simulink model "first_gear_model_non_linear"  (R2020b)
settings: Solver=FixedStepAuto  StartTime=0.0  StopTime=5  FixedStep=0.0001  RelTol=1e-3
settings Model: Creator=morro  LastModifiedBy=morro

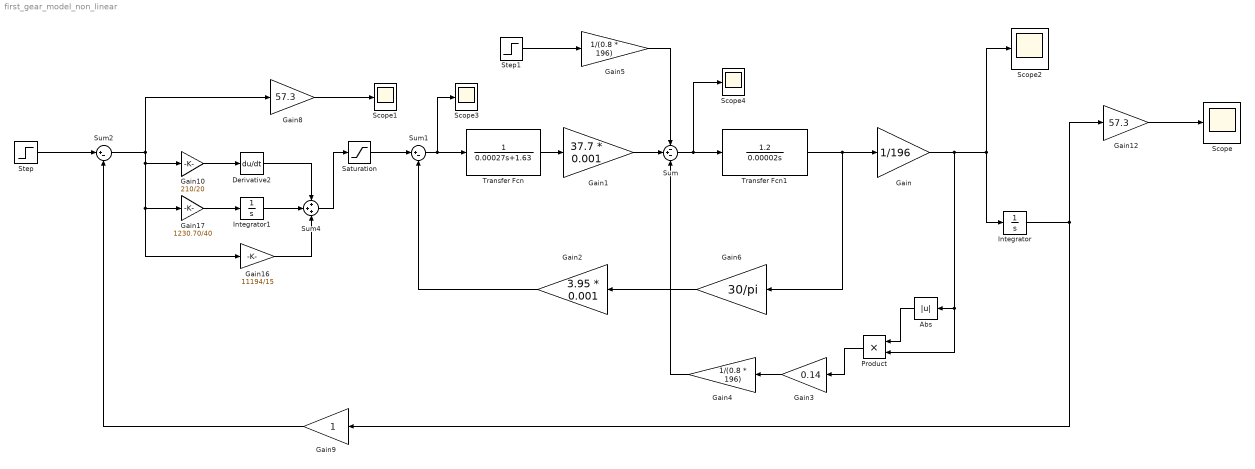
== system first_gear_model_non_linear ==
  Abs : Abs
  Derivative2 : Derivative
  Gain : Gain  Gain=1/196
  Gain1 : Gain  Gain=37.7 * 0.001
  Gain10 : Gain  Gain=210/20
  Gain12 : Gain  Gain=57.3
  Gain16 : Gain  Gain=11194/15
  Gain17 : Gain  Gain=1230.70/40
  Gain2 : Gain  Gain=3.95 * 0.001
  Gain3 : Gain  Gain=0.14
  Gain4 : Gain  Gain=1/(0.8 * 196)
  Gain5 : Gain  Gain=1/(0.8 * 196)
  Gain6 : Gain  Gain=30/pi
  Gain8 : Gain  Gain=57.3
  Gain9 : Gain
  Integrator : Integrator  InitialCondition=1e-7
  Integrator1 : Integrator  InitialCondition=1e-7
  Product : Product
  Saturation : Saturate  UpperLimit=27  LowerLimit=-27
  Scope{,1..4} (5 alike) : Scope
  Step : Step  After=100/57.3  SampleTime=0
  Step1 : Step  Time=2  After=9  SampleTime=0
  Sum : Sum  Inputs=-+-
  Sum1 : Sum  Inputs=|+-
  Sum2 : Sum  Inputs=|+-
  Sum4 : Sum  Inputs=+++
  Transfer Fcn : TransferFcn  Denominator=[0.00027 1.63]
  Transfer Fcn1 : TransferFcn  Numerator=[1.2]  Denominator=[0.00002 0]
  wires:
  Gain/1 -> Product/2, Abs/1, Integrator/1, Scope2/1
  Gain3/1 -> Gain4/1
  Gain9/1 -> Sum2/2
  Transfer Fcn/1 -> Gain1/1
  Integrator1/1 -> Sum4/2
  Gain17/1 -> Integrator1/1
  Gain2/1 -> Sum1/2
  Abs/1 -> Product/1
  Gain12/1 -> Scope/1
  Sum2/1 -> Gain16/1, Gain17/1, Gain10/1, Gain8/1
  Derivative2/1 -> Sum4/1
  Gain5/1 -> Sum/1
  Gain8/1 -> Scope1/1
  Step/1 -> Sum2/1
  Gain6/1 -> Gain2/1
  Transfer Fcn1/1 -> Gain6/1, Gain/1
  Step1/1 -> Gain5/1
  Gain1/1 -> Sum/2
  Gain16/1 -> Sum4/3
  Gain10/1 -> Derivative2/1
  Gain4/1 -> Sum/3
  Sum/1 -> Scope4/1, Transfer Fcn1/1
  Integrator/1 -> Gain9/1, Gain12/1
  Product/1 -> Gain3/1
  Saturation/1 -> Sum1/1
  Sum1/1 -> Scope3/1, Transfer Fcn/1
  Sum4/1 -> Saturation/1
